simulink library "sensors_T2_lib"  (Simulink 7.2)
settings: Solver=ode45  SolverMode=SingleTasking  StartTime=0.0  StopTime=10.0  RelTol=1e-3
undefined symbols (not defined in the file or in its folder): alphavl_offset, alphavl_pos, alphavl_upwash, alphavr_offset, alphavr_pos, alphavr_upwash, betavl_offset, betavl_pos, betavl_sidewash, betavr_offset, betavr_pos, betavr_sidewash, POS_hi, POS_lo, Timestep
libraries: aeroutilslib x19, NoiseModel_lib x9, simulink_extras x6, SignalConditioning_lib x2, Latency_lib x1, sensor_failure_lib x1, simulink x1
(part 2 of 2)

== system sensors_T2_lib/GTM_T2/MIDG II 50 Hz/Port 3, MIDG Data/STATUS MSG ID 1 ==
  note: Current Mode
      | IMU: Inertial Measuring Unit
      | VG:  Vertical Gyro
      | INS: Inertial Navigation System
      |
      | 1=IMU
      | 2=VG INIT
      | 3=VG FAST
      | 4=VG MEDIUM
      | 5=VG SLOW
      | 6=VG SE
      | 7=INS
  Clock : Clock
      settings: Decimation=10
  Constant{,1..2,4} (4 alike) : Constant  Value=0  OutDataType=sfix(16)  OutScaling=2^0
  Constant3 : Constant  Value=7  OutDataType=sfix(16)  OutScaling=2^0
  TimeStamp : Outport  OutDataType=sfix(16)  OutScaling=2^0
  NV_config_inv : Outport  Port=2  OutDataType=sfix(16)  OutScaling=2^0
  GPS_time_valid : Outport  Port=3  OutDataType=sfix(16)  OutScaling=2^0
  DGPS : Outport  Port=4  OutDataType=sfix(16)  OutScaling=2^0
  mode : Outport  Port=5  OutDataType=sfix(16)  OutScaling=2^0
  temperature : Outport  Port=6  OutDataType=sfix(16)  OutScaling=2^0
  wires:
  Constant4/1 -> temperature/1  "int_temperature"
  Constant3/1 -> mode/1  "MIDG_mode"
  Constant2/1 -> DGPS/1  "DGPS"
  Constant1/1 -> GPS_time_valid/1  "GPS_time_valid"
  Constant/1 -> NV_config_inv/1  "NV_config_inv"
  Clock/1 -> TimeStamp/1  "GPS_TIME"

== system sensors_T2_lib/GTM_T2/MIDG II 50 Hz/Port 3, MIDG Data/TIM_ERR MSG ID 26 ==
  Clock : Clock
      settings: Decimation=10
  Constant1 : Constant  Value=0  OutDataType=sfix(16)  OutScaling=2^0
  Constant2 : Constant  Value=0  OutDataType=sfix(16)  OutScaling=2^0
  Constant3 : Constant  Value=0  OutDataType=sfix(16)  OutScaling=2^0
  TimeStamp : Outport  OutDataType=sfix(16)  OutScaling=2^0
  TTB : Outport  Port=2  OutDataType=sfix(16)  OutScaling=2^0
  DTB : Outport  Port=3  OutDataType=sfix(16)  OutScaling=2^0
  flags : Outport  Port=4  OutDataType=sfix(16)  OutScaling=2^0
  wires:
  Constant3/1 -> flags/1  "GPS_TimErr_flags"
  Constant2/1 -> DTB/1  "GPS_DTB"
  Constant1/1 -> TTB/1  "GPS_TTB"
  Clock/1 -> TimeStamp/1  "GPS_TIME"

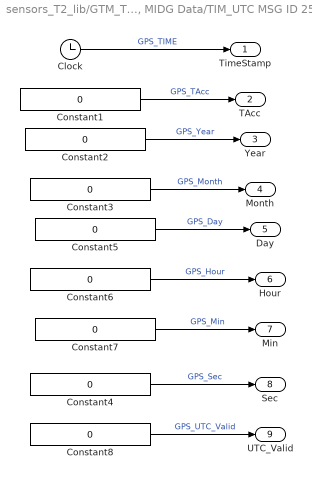
== system sensors_T2_lib/GTM_T2/MIDG II 50 Hz/Port 3, MIDG Data/TIM_UTC MSG ID 25 ==
  Clock : Clock
      settings: Decimation=10
  Constant{1..8} (8 alike) : Constant  Value=0  OutDataType=sfix(16)  OutScaling=2^0
  TimeStamp : Outport  OutDataType=sfix(16)  OutScaling=2^0
  TAcc : Outport  Port=2  OutDataType=sfix(16)  OutScaling=2^0
  Year : Outport  Port=3  OutDataType=sfix(16)  OutScaling=2^0
  Month : Outport  Port=4  OutDataType=sfix(16)  OutScaling=2^0
  Day : Outport  Port=5  OutDataType=sfix(16)  OutScaling=2^0
  Hour : Outport  Port=6  OutDataType=sfix(16)  OutScaling=2^0
  Min : Outport  Port=7  OutDataType=sfix(16)  OutScaling=2^0
  Sec : Outport  Port=8  OutDataType=sfix(16)  OutScaling=2^0
  UTC_Valid : Outport  Port=9  OutDataType=sfix(16)  OutScaling=2^0
  wires:
  Constant8/1 -> UTC_Valid/1  "GPS_UTC_Valid"
  Constant7/1 -> Min/1  "GPS_Min"
  Constant6/1 -> Hour/1  "GPS_Hour"
  Constant5/1 -> Day/1  "GPS_Day"
  Constant3/1 -> Month/1  "GPS_Month"
  Constant2/1 -> Year/1  "GPS_Year"
  Constant1/1 -> TAcc/1  "GPS_TAcc"
  Constant4/1 -> Sec/1  "GPS_Sec"
  Clock/1 -> TimeStamp/1  "GPS_TIME"

== system sensors_T2_lib/GTM_T2/MIDG II 50 Hz/Port 3, MIDG Data/IMU_DATA MSG ID 2/Subsystem3 ==
  I : Inport  OutDataType=sfix(16)  OutScaling=2^0
  Constant1 : Constant  Value=2*pi  OutDataType=sfix(16)  OutScaling=2^0
  Constant2 : Constant  Value=2*pi  OutDataType=sfix(16)  OutScaling=2^0
  Constant3 : Constant  Value=2*pi  OutDataType=sfix(16)  OutScaling=2^0
  Math Function1 : Math  Operator=rem  OutDataType=sfix(16)  OutScaling=2^0  SaturateOnIntegerOverflow=on
  Sum : Sum  Inputs=|-+  OutDataType=sfix(16)  OutScaling=2^0  SaturateOnIntegerOverflow=on
  Sum1 : Sum  Inputs=++|  OutDataType=sfix(16)  OutScaling=2^0  SaturateOnIntegerOverflow=on
  Switch : Switch  Criteria=u2 > Threshold  Threshold=pi  SaturateOnIntegerOverflow=on
  Switch1 : Switch  SaturateOnIntegerOverflow=on
  Switch2 : Switch  Threshold=-pi  SaturateOnIntegerOverflow=on
  O : Outport  OutDataType=sfix(16)  OutScaling=2^0
  wires:
  Constant1/1 -> Math Function1/2
  I/1 -> Math Function1/1
  Math Function1/1 -> Switch/2, Sum/2, Switch/3, Switch2/1, Switch2/2, Sum1/1, Switch1/2
  Constant2/1 -> Sum/1
  Sum/1 -> Switch/1
  Constant3/1 -> Sum1/2
  Sum1/1 -> Switch2/3
  Switch2/1 -> Switch1/3
  Switch/1 -> Switch1/1
  Switch1/1 -> O/1

== system sensors_T2_lib/GTM_T2/MIDG II 50 Hz/Port 3, MIDG Data/IMU_MAG MSG ID 3/Subsystem3 ==
  I : Inport  OutDataType=sfix(16)  OutScaling=2^0
  Constant1 : Constant  Value=2*pi  OutDataType=sfix(16)  OutScaling=2^0
  Constant2 : Constant  Value=2*pi  OutDataType=sfix(16)  OutScaling=2^0
  Constant3 : Constant  Value=2*pi  OutDataType=sfix(16)  OutScaling=2^0
  Math Function1 : Math  Operator=rem  OutDataType=sfix(16)  OutScaling=2^0  SaturateOnIntegerOverflow=on
  Sum : Sum  Inputs=|-+  OutDataType=sfix(16)  OutScaling=2^0  SaturateOnIntegerOverflow=on
  Sum1 : Sum  Inputs=++|  OutDataType=sfix(16)  OutScaling=2^0  SaturateOnIntegerOverflow=on
  Switch : Switch  Criteria=u2 > Threshold  Threshold=pi  SaturateOnIntegerOverflow=on
  Switch1 : Switch  SaturateOnIntegerOverflow=on
  Switch2 : Switch  Threshold=-pi  SaturateOnIntegerOverflow=on
  O : Outport  OutDataType=sfix(16)  OutScaling=2^0
  wires:
  Constant1/1 -> Math Function1/2
  I/1 -> Math Function1/1
  Math Function1/1 -> Switch/2, Sum/2, Switch/3, Switch2/1, Switch2/2, Sum1/1, Switch1/2
  Constant2/1 -> Sum/1
  Sum/1 -> Switch/1
  Constant3/1 -> Sum1/2
  Sum1/1 -> Switch2/3
  Switch2/1 -> Switch1/3
  Switch/1 -> Switch1/1
  Switch1/1 -> O/1

== system sensors_T2_lib/GTM_T2/MIDG II 50 Hz/Port 3, MIDG Data/NAV_SENSOR MSG ID 10/Subsystem3 ==
  I : Inport  OutDataType=sfix(16)  OutScaling=2^0
  Constant : Constant  Value=0  OutDataType=sfix(16)  OutScaling=2^0
  Constant4 : Constant  Value=360  OutDataType=sfix(16)  OutScaling=2^0
  Sum2 : Sum  Inputs=|+-  OutDataType=sfix(16)  OutScaling=2^0  SaturateOnIntegerOverflow=on
  Switch3 : Switch  Threshold=180  SaturateOnIntegerOverflow=on
  O : Outport  OutDataType=sfix(16)  OutScaling=2^0
  wires:
  I/1 -> Switch3/2, Sum2/1
  Sum2/1 -> O/1
  Switch3/1 -> Sum2/2
  Constant/1 -> Switch3/3
  Constant4/1 -> Switch3/1

== system sensors_T2_lib/GTM_T2/MIDG II 50 Hz/Port 3, MIDG Data/NAV_SENSOR MSG ID 10/quaternion ==
  Euler angles : Inport  OutDataType=sfix(16)  OutScaling=2^0
  1/2 : Gain  Gain=1/2  ParameterDataType=sfix(16)  ParameterScaling=2^0  OutDataType=sfix(16)  OutScaling=2^0  SaturateOnIntegerOverflow=on  OutDataTypeStr=Inherit: Same as input  ParamDataTypeStr=Inherit: Same as input
  Cos(Euler/2) : Trigonometry  Operator=cos
  Mux1 : Mux  Inputs=2
  Mux2 : Mux
  Sin(Euler/2) : Trigonometry
  e0 : Fcn  Expr=u(1)*u(2)*u(3)+u(4)*u(5)*u(6)
  e1 : Fcn  Expr=-u(2)*u(3)*u(4)+u(1)*u(5)*u(6)
  e2 : Fcn  Expr=u(1)*u(5)*u(3)+u(2)*u(4)*u(6)
  e3 : Fcn  Expr=u(3)*u(4)*u(5)-u(1)*u(2)*u(6)
  Quaternions : Outport  OutDataType=sfix(16)  OutScaling=2^0
  wires:
  1/2/1 -> Sin(Euler/2)/1, Cos(Euler/2)/1
  Sin(Euler/2)/1 -> Mux1/1
  Cos(Euler/2)/1 -> Mux1/2
  Mux1/1 -> e2/1, e3/1, e1/1, e0/1
  e0/1 -> Mux2/1
  e1/1 -> Mux2/2
  e2/1 -> Mux2/3
  e3/1 -> Mux2/4
  Euler angles/1 -> 1/2/1
  Mux2/1 -> Quaternions/1

== matlab function GTM_T2/MAG3 IMU/Embedded MATLAB Function ==
  data: omega input double; omega_dot input double; cg_pos input double; nbody input double; n_body output double; MAG3_pos parameter double
function n_body = accel_model(omega,omega_dot,cg_pos,nbody,MAG3_pos)
% Compute off-CG accelerometer corrections.  
% Inputs:
%       omega: body-axis angular rates, [p q r], in rad/sec

%   omega_dot: body-axis angular accelerations, [pdot qdot rdot], rad/sec^2
%       nbody: body-axis accels at CG [Nx Ny Nz], g
%      cg_pos: cg position, feet
%   MAG3_pos: accelerometer position, feet
%
% Note: cg and accel position must be in the same reference frame
%
% Author: Austin Murch (Austin.M.Murch@nasa.gov)
% Created: 11-2-2007

g0    = 32.174;

cg2accel = MAG3_pos' - cg_pos;

n_body =  nbody + (cross(omega,cross(omega,cg2accel)) + cross(omega_dot,cg2accel))/g0;

== matlab function GTM_T2/MIDG II 50 Hz/ENU to ECEF ==
  data: u input double; y output double
function y = fcn(u)
% Convert ENU position/velocity to ECEF, output both.

y = zeros(1,12); % initialize output length
 
d2r = pi/180; 
Vn  = u(1);
Ve  = u(2);
Vu  = u(3);
lat = u(4)*d2r;
lon = u(5)*d2r;
alt = u(6);

a2 = 4.068063159076900e+013; %m^2, Earth ellipsoid major axis squared
b2 = 4.040829998408706e+013; %m^2, Earth ellipsoid minor axis squared

N = a2/sqrt(a2*cos(lat)^2 + b2*sin(lat)^2);

XE = (alt + N)*cos(lat)*cos(lon);
YE = (alt + N)*cos(lat)*sin(lon);
ZE = (alt + N)*b2/a2*sin(lat);

VXE = Ve*sin(lat)*cos(lat) - Vn*sin(lon) - Vu*sin(lat)*cos(lon);
VYE = Ve*cos(lat)*sin(lon) + Vn*cos(lon) - Vu*sin(lat)*sin(lon);
VZE = Ve*sin(lat) + Vu*cos(lat);


y = [lat/d2r lon/d2r alt Vn Ve Vu XE YE ZE VXE VYE VZE];

== matlab function GTM_T2/MIDG II 50 Hz/Embedded MATLAB Function ==
  data: omega input double; omega_dot input double; cg_pos input double; nbody input double; n_body output double; MIDG_pos parameter double
function n_body = accel_model(omega,omega_dot,cg_pos,nbody,MIDG_pos)
% Compute off-CG accelerometer corrections.  
% Inputs:
%       omega: body-axis angular rates, [p q r], in rad/sec

%   omega_dot: body-axis angular accelerations, [pdot qdot rdot], rad/sec^2
%       nbody: body-axis accels at CG [Nx Ny Nz], g
%      cg_pos: cg position, feet
%    MIDG_pos: accelerometer position, feet
%
% Note: cg and accel position must be in the same reference frame
%
% Author: Austin Murch (Austin.M.Murch@nasa.gov)
% Created: 11-2-2007

g0    = 32.174;

cg2accel = MIDG_pos' - cg_pos;

n_body =  nbody + (cross(omega,cross(omega,cg2accel)) + cross(omega_dot,cg2accel))/g0;

== matlab function GTM_T2/Vanes/Embedded MATLAB Function ==
  data: omega input double; alphavl output double; alpha input double; beta input double; vt input double; betavl output double; alphavr output double; betavr output double; cg_pos input double; alphavl_pos parameter double; alphavl_offset parameter double; alphavr_pos parameter double; alphavr_offset parameter double; betavl_pos parameter double; betavl_offset parameter double; betavr_pos parameter double; betavr_offset parameter double; alphavl_upwash parameter double; alphavr_upwash parameter double; betavl_sidewash parameter double; betavr_sidewash parameter double
function [alphavl,betavl,alphavr,betavr] = vane_model(omega,alpha,beta,vt,cg_pos,...
                                                      alphavl_pos,alphavl_offset,alphavr_pos,alphavr_offset,...
                                                      betavl_pos,betavl_offset,betavr_pos,betavr_offset,...
                                                      alphavl_upwash,alphavr_upwash,betavl_sidewash,betavr_sidewash)
% This block supports the Embedded MATLAB subset.
% See the help menu for details.

r2d       = 180/pi;         % nd      multiply radians by this to get degress
kts2fps   = 1.6889;         % nd      multiply knots by this to get fps

% prevent divide by zero
if vt < 1
    vt = 1;
end

% CG to vane position
cg2alphavl = alphavl_pos' - cg_pos;
cg2alphavr = alphavr_pos' - cg_pos;
cg2betavl  = betavl_pos' - cg_pos;
cg2betavr  = betavr_pos' - cg_pos;

% Alpha/Beta vane models

% Alpha/Beta upwash/sidewash corrections
alphavrc = interp1(alphavr_upwash(1,:),alphavr_upwash(2,:),alpha,'linear','extrap');
alphavlc = interp1(alphavl_upwash(1,:),alphavl_upwash(2,:),alpha,'linear','extrap');
betavrc  = interp1(betavr_sidewash(1,:),betavr_sidewash(2,:),beta,'linear','extrap');
betavlc  = interp1(betavl_sidewash(1,:),betavl_sidewash(2,:),beta,'linear','extrap');

% Add boom alignment errors and angular rate corrections
alphavr  =  (alphavrc - r2d.*(omega(2).*cg2alphavr(1) - omega(1).*cg2alphavr(2))./(vt.*kts2fps) - alphavr_offset);
alphavl  =  (alphavlc - r2d.*(omega(2).*cg2alphavl(1) - omega(1).*cg2alphavl(2))./(vt.*kts2fps) - alphavl_offset);
betavr   =  (betavrc - r2d.*(omega(1).*cg2betavr(3) - omega(3).*cg2betavr(1))./(vt.*kts2fps) - betavr_offset);
betavl  =  (betavlc - r2d.*(omega(1).*cg2betavl(3) - omega(3).*cg2betavl(1))./(vt.*kts2fps) - betavl_offset);
